simulink model "t06_manual_control"  (R2024b)
settings: Solver=ode23t  StartTime=0.0  StopTime=inf  RelTol=1e-3  AbsTol=1e-3  EnableMultiTasking=on
model workspace (MAT data in the model file):
  A = 0.4
  Critical_Velocity = 0.01
  Damping_Factor = 1000
  Dynamic_Friction = 0.5
  Heigth_brick : Simulink.Parameter (value not decoded)
  Heigth_ramp : Simulink.Parameter (value not decoded)
  Length_brick : Simulink.Parameter (value not decoded)
  Length_ramp : Simulink.Parameter (value not decoded)
  Length_torso : Simulink.Parameter (value not decoded)
  Lower_limbs : Simulink.Parameter (value not decoded)
  Static_Friction = 0.7
  Stiffnesscoefficient = 10000
  Transition_Region_Width = 0.02
  Upper_limbs : Simulink.Parameter (value not decoded)
  Width_brick : Simulink.Parameter (value not decoded)
  Width_ramp : Simulink.Parameter (value not decoded)
  Width_torso : Simulink.Parameter (value not decoded)
  f = 1.5
  max_Joint_change = 100
  r_foot : Simulink.Parameter (value not decoded)
  sampleTime : Simulink.Parameter (value not decoded)
  t_leg : Simulink.Parameter (value not decoded)
  theta : Simulink.Parameter (value not decoded)
  transferFunVal : Simulink.Parameter (value not decoded)
symbols that are objects in the model workspace (value not decoded): Length_torso, Lower_limbs, t_leg, Upper_limbs, Width_torso
undefined symbols (not defined in the file): X, Y, Z
libraries: sm_lib x78, nesl_utility x13, functionAngles x6, functionBezier_backward x3, vrlib x1
(part 5 of 5)

== matlab function t06_manual_control/WALK FORWARD GAIT/Plane Movement Forward/MATLAB Function2 ==
  data: x output; t input; Tdur input; y output; P0x input; P0z input; P1x input; P1z input; P2x input; P2z input; P3x input; P3z input
function [x, y] = bez_plane_TrajV2(t,Tdur,P0x,P0z,P1x,P1z,P2x,P2z,P3x,P3z)
t_swing = Tdur/4;
t_support = Tdur*3/4;

P0 = [P0x, P0z];
P1 = [P1x, P1z];
P2 = [P2x, P2z];
P3 = [P3x, P3z];
P_ini = (P0 + P3)/2;

if Tdur == 0
    x = -P_ini(1);
    y = P_ini(2);

elseif t<=t_support/2
    x = -1*(P_ini(1)+(P0(1)-P3(1))/t_support*(t));
    y = P_ini(2);

elseif t<=t_support/2+t_swing
    t_ef = (t-t_support/2);
    Sw = P0*((1-(t_ef/t_swing))^3) + 3*P1*(t_ef/t_swing)*((1-(t_ef/t_swing))^2)...
        + 3*P2*((t_ef/t_swing)^2)*(1-(t_ef/t_swing)) + P3*((t_ef/t_swing)^3);
    
    x = -1*Sw(1);
    y = Sw(2);
else
    t_ef = (t-t_support/2-t_swing);
    x = -1*(P3(1)+(P0(1)-P3(1))/t_support*t_ef);
    y = P0(2);
end

end

== matlab function t06_manual_control/TURN RIGHT GAIT/Plane Movement Left1/MATLAB Function ==
  data: x input; theta1Ad output; L1 input; L2 input; theta1 input
function theta1Ad = angAd(x, L1, L2, theta1)

l = cos(theta1)*(L1 + L2);

theta1Ad = asin(-x/l);
